simulink model "Current"  (R2022b)
settings: Solver=VariableStepAuto  StartTime=0.0  StopTime=inf  RelTol=1e-3
libraries: slDxl_lib x8
settings Model: Creator=jeihunl  LastModifiedBy=Boog
settings SolverCC: AlgebraicLoopSolver=TrustRegion
settings DataIOCC: ReturnWorkspaceOutputs=off
settings DebuggingCC: UnconnectedInputMsg=warning  UnconnectedOutputMsg=warning  UnconnectedLineMsg=warning  SFMachineParentedDataDiag=warning  ArithmeticOperatorsInVariantConditions=warning
settings ModelReferenceCC: EnableRefExpFcnMdlSchedulingChecks=on
settings SFSimCC: SimUseLocalCustomCode=off  CustomCodeUndefinedFunction=UseInterfaceOnly
settings RTWCC: RTWUseLocalCustomCode=off
settings CodeAppCC: StateflowObjectComments=on

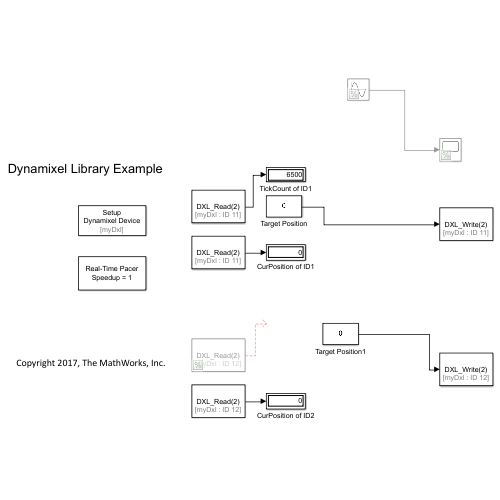
[thumbnail: Simulink's stored preview of the top-level diagram]
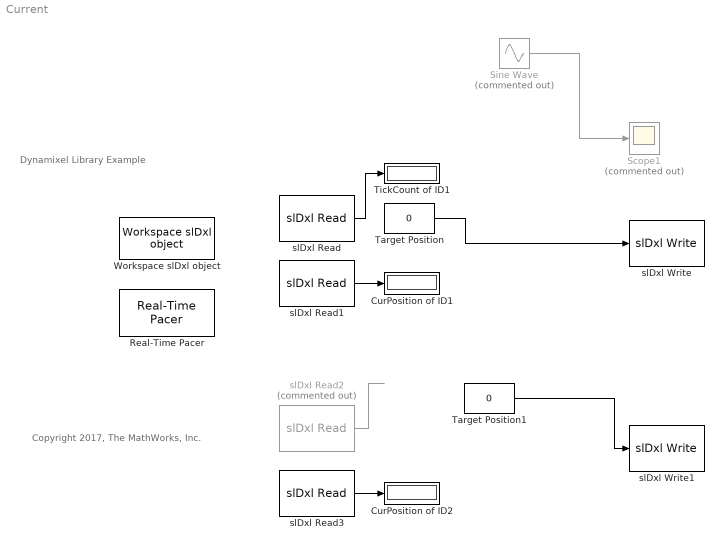
== system Current ==
  note: Dynamixel Library Example
  note: Copyright 2017, The MathWorks, Inc.
  CurPosition of ID1 : Display
  CurPosition of ID2 : Display
  Real-Time Pacer : slDxl_lib/Real-Time Pacer  simTimePerRealTime=1
  Scope1 : Scope  Commented=on
  Sine Wave : Sin  Commented=on  Amplitude=100  SampleTime=0
  Target Position : Constant  Value=0  OutDataTypeStr=int16
  Target Position1 : Constant  Value=0  OutDataTypeStr=int16
  TickCount of ID1 : Display
  Workspace slDxl object : slDxl_lib/Workspace slDxl object  slDxlVarName=Existing Object Handle #1  workspaceVarName=myDxl
  slDxl Read : slDxl_lib/slDxl Read  slDxlObject=Existing Object Handle #1  DXL_ID=11  DXL_ADDR=120  DXL_READ_SIZE=2  sampleT=Ts
  slDxl Read1 : slDxl_lib/slDxl Read  slDxlObject=Existing Object Handle #1  DXL_ID=11  DXL_ADDR=126  DXL_READ_SIZE=2  sampleT=Ts
  slDxl Read2 : slDxl_lib/slDxl Read  Commented=on  slDxlObject=Existing Object Handle #1  DXL_ID=12  DXL_ADDR=120  DXL_READ_SIZE=2  sampleT=Ts
  slDxl Read3 : slDxl_lib/slDxl Read  slDxlObject=Existing Object Handle #1  DXL_ID=12  DXL_ADDR=126  DXL_READ_SIZE=2  sampleT=Ts
  slDxl Write : slDxl_lib/slDxl Write  slDxlObject=Existing Object Handle #1  DXL_ID=11  DXL_ADDR=102  DXL_WRITE_SIZE=2  sampleT=Ts
  slDxl Write1 : slDxl_lib/slDxl Write  slDxlObject=Existing Object Handle #1  DXL_ID=12  DXL_ADDR=102  DXL_WRITE_SIZE=2  sampleT=Ts
  wires:
  slDxl Read/1 -> TickCount of ID1/1
  slDxl Read1/1 -> CurPosition of ID1/1
  slDxl Read2/1 -> ?
  Target Position1/1 -> slDxl Write1/1
  slDxl Read3/1 -> CurPosition of ID2/1
  Sine Wave/1 -> Scope1/1
  Target Position/1 -> slDxl Write/1
